simulink subsystem "subsys_calcul_Zk_2021A"  (R2021a)
settings: Solver=VariableStepAuto  StartTime=0.0  StopTime=10.0  RelTol=1e-3
settings Model: Creator=antho  LastModifiedBy=alexi

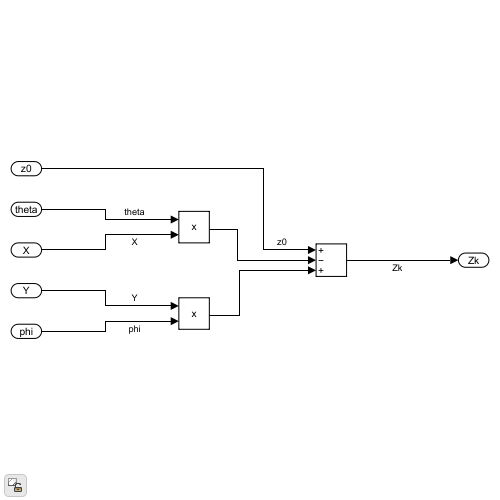
[thumbnail: Simulink's stored preview of the top-level diagram]
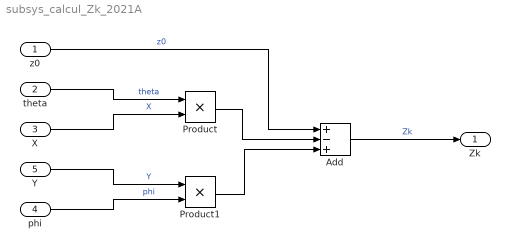
== system subsys_calcul_Zk_2021A ==
  z0 : Inport
  theta : Inport  Port=2
  X : Inport  Port=3
  phi : Inport  Port=4
  Y : Inport  Port=5
  Add : Sum  Inputs=+-+
  Product : Product
  Product1 : Product
  Zk : Outport
  wires:
  phi/1 -> Product1/2  "phi"
  theta/1 -> Product/1  "theta"
  X/1 -> Product/2  "X"
  z0/1 -> Add/1  "z0"
  Y/1 -> Product1/1  "Y"
  Product/1 -> Add/2
  Product1/1 -> Add/3
  Add/1 -> Zk/1  "Zk"
